simulink subsystem "PWM"  (R2020b)
settings: Solver=VariableStepAuto  StartTime=0.0  StopTime=10.0  RelTol=1e-3
undefined symbols (not defined in the file): T_sim
settings Model: Creator=leop9  LastModifiedBy=Previ

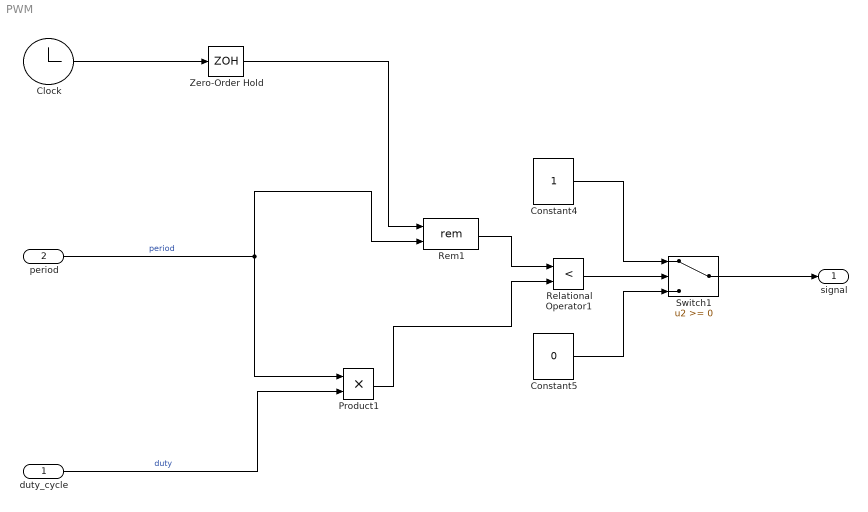
== system PWM ==
  duty_cycle : Inport
  period : Inport  Port=2
  Clock : Clock
  Constant4 : Constant  OutDataTypeStr=double
  Constant5 : Constant  Value=0  OutDataTypeStr=double
  Product1 : Product
  Relational Operator1 : RelationalOperator  Operator=<  OutDataTypeStr=boolean  RndMeth=Ceiling
  Rem1 : Math  Operator=rem  SaturateOnIntegerOverflow=on
  Switch1 : Switch
  Zero-Order Hold : ZeroOrderHold  SampleTime=T_sim
  signal : Outport
  wires:
  Product1/1 -> Relational Operator1/2
  Zero-Order Hold/1 -> Rem1/1
  period/1 -> Rem1/2, Product1/1  "period"
  duty_cycle/1 -> Product1/2  "duty"
  Switch1/1 -> signal/1
  Rem1/1 -> Relational Operator1/1
  Clock/1 -> Zero-Order Hold/1
  Constant5/1 -> Switch1/3
  Relational Operator1/1 -> Switch1/2
  Constant4/1 -> Switch1/1
